simulink model "draft7"  (R2023a)
settings: Solver=VariableStepAuto  StartTime=0.0  StopTime=10  FixedStep=0.0001  MaxStep=0.1  RelTol=1e-3  AbsTol=1e-3  EnableMultiTasking=on
model workspace (MAT data in the model file):
  C_Gimbal = 0.1
  C_IAP = 0.01
  IAP_Pa = 0
  K_Gimbal = 0
  K_IAP = 10
  LeftAbdominalMuscleForce = 0
  LeftBackMuscleForce = 0
  LeftTransverse1MuscleForce = 0
  LeftTransverse2MuscleForce = 0
  Moment_AR = 0
  Moment_FE = 0
  Moment_LB = 0
  RightAbdominalMuscleForce = 0
  RightBackMuscleForce = 0
  RightTransverse1MuscleForce = 0
  RightTransverse2MuscleForce = 0
  a = 1
  b = 1
undefined symbols (not defined in the file): X, Y, Z
libraries: sm_lib x279, nesl_utility x233, simulink_extras x33, checkpacklib x3, simulink x1
(part 5 of 7)

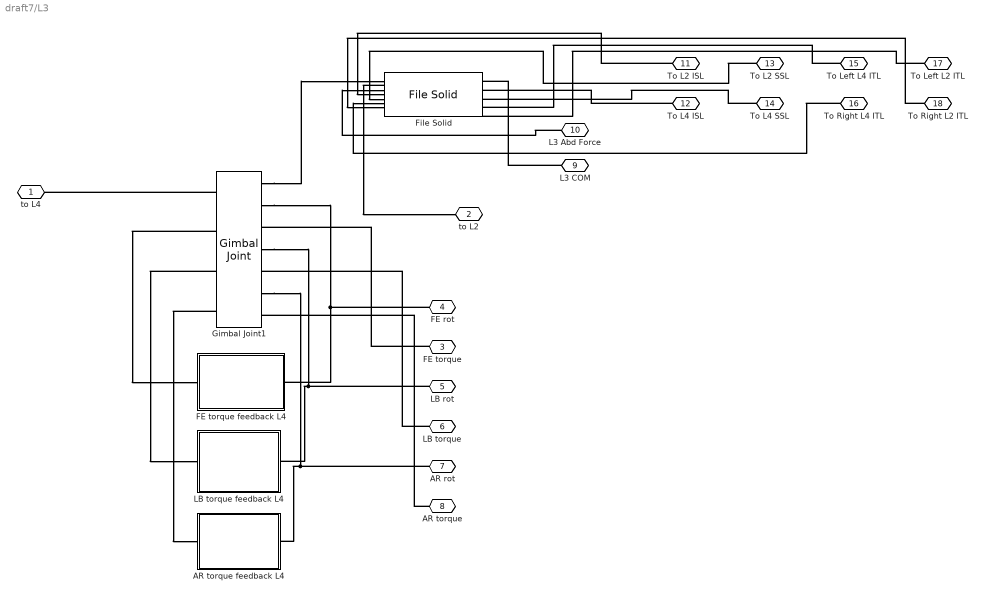
== system draft7/L3 ==
  AR torque feedback L4 : Subsystem
  FE torque feedback L4 : Subsystem
  File Solid : sm_lib/Body Elements/File Solid  ExtGeomFileName=C:\Users\siril\OneDrive\Desktop\TIM-Control\Matlab\Simscape models\CAD - with COM\SymmetricModel\draft7\L3.step  UnitType=FromFile  ExtGeomFileUnits=m  StepReaderType=HEX  ExportConvexHullGeometry=off  InertiaType=CalculateFromGeometry  Mass=1  MassUnits=kg  CenterOfMass=[0 0 0]  CenterOfMassUnits=m  MomentsOfInertia=[1 1 1]  MomentsOfInertiaUnits=kg*m^2  ProductsOfInertia=[0 0 0]  ProductsOfInertiaUnits=kg*m^2  BasedOnType=Density  Density=0.182  DensityUnits=g/cm^3  DoExposeReferenceFrame=on  SerializedFrames=<Frames><Frame><Id>Frame1</Id><Value><Name>To L4</Name><Origin><Source>GeometricFeature</Source><FeatureName>planar surface 3165</FeatureName></Origin><PrimaryAxis><DefinedDirection>+Z</DefinedDirection><Source>GeometricFeature</Source><SourceDirection>+Z</SourceDirection><FeatureName>planar surface 3165</FeatureName></PrimaryAxis><SecondaryAxis><DefinedDirection>+X</DefinedDirection><Source>ReferenceFrame</Source><SourceDirection>+X</SourceDirection><FeatureName></FeatureName></SecondaryAxis></Value></Frame><Frame><Id>Frame2</Id><Value><Name>To L2</Name><Origin><Source>GeometricFeature</Source><FeatureName>planar surface 3181</FeatureName></Origin><PrimaryAxis><DefinedDirection>+Z</DefinedDirection><Source>GeometricFeature</Source><SourceDirection>+Z</SourceDirection><FeatureName>planar surface 3181</FeatureName></PrimaryAxis><SecondaryAxis><DefinedDirection>+X</DefinedDirection><Source>ReferenceFrame</Source><SourceDirection>+X</SourceDirection><FeatureName></FeatureName></SecondaryAxis></Value></Frame><Frame><Id>Frame3</Id><Value><Name>L3 COM</Name><Origin><Source>CenterOfMassFrame</Source><FeatureName></FeatureName></Origin><PrimaryAxis><DefinedDirection>+Z</DefinedDirection><Source>ReferenceFrame</Source><SourceDirection>+Z</SourceDirection><FeatureName></FeatureName></PrimaryAxis><SecondaryAxis><DefinedDirection>+X</DefinedDirection><Source>ReferenceFrame</Source><SourceDirection>+X</SourceDirection><FeatureName></FeatureName></SecondaryAxis></Value></Frame><Frame><Id>Frame4</Id><Value><Name>L3 Abd Force</Name><Origin><Source>GeometricFeature</Source><FeatureName>point 3</FeatureName></Origin><PrimaryAxis><DefinedDirection>+Z</DefinedDirection><Source>GeometricFeature</Source><SourceDirection>+Z</SourceDirection><FeatureName>conical surface 2</FeatureName></PrimaryAxis><SecondaryAxis><DefinedDirection>+X</DefinedDirection><Source>ReferenceFrame</Source><SourceDirection>+X</SourceDirection><FeatureName></FeatureName></SecondaryAxis></Value></Frame><Frame><Id>Frame5</Id><Value><Name>To L4 ISL</Name><Origin><Source>GeometricFeature</Source><FeatureName>point 6019</FeatureName></Origin><PrimaryAxis><DefinedDirection>+Z</DefinedDirection><Source>ReferenceFrame</Source><SourceDirection>+Z</SourceDirection><FeatureName></FeatureName></PrimaryAxis><SecondaryAxis><DefinedDirection>+X</DefinedDirection><Source>ReferenceFrame</Source><SourceDirection>+X</SourceDirection><FeatureName></FeatureName></SecondaryAxis></Value></Frame><Frame><Id>Frame6</Id><Value><Name>To L2 ISL</Name><Origin><Source>GeometricFeature</Source><FeatureName>segment 2486</FeatureName></Origin><PrimaryAxis><DefinedDirection>+Z</DefinedDirection><Source>ReferenceFrame</Source><SourceDirection>+Z</SourceDirection><FeatureName></FeatureName></PrimaryAxis><SecondaryAxis><DefinedDirection>+X</DefinedDirection><Source>ReferenceFrame</Source><SourceDirection>+X</SourceDirection><FeatureName></FeatureName></SecondaryAxis></Value></Frame><Frame><Id>Frame7</Id><Value><Name>To L4 SSL</Name><Origin><Source>GeometricFeature</Source><FeatureName>point 5053</FeatureName></Origin><PrimaryAxis><DefinedDirection>+Z</DefinedDirection><Source>ReferenceFrame</Source><SourceDirection>+Z</SourceDirection><FeatureName></FeatureName></PrimaryAxis><SecondaryAxis><DefinedDirection>+X</DefinedDirection><Source>ReferenceFrame</Source><SourceDirection>+X</SourceDirection><FeatureName></FeatureName></SecondaryAxis></Value></Frame><Frame><Id>Frame8</Id><Value><Name>To L2 SSL</Name><Origin><Source>GeometricFeature</Source><FeatureName>point 5046</FeatureName></Origin><PrimaryAxis><DefinedDirection>+Z</DefinedDirection><Source>ReferenceFrame</Source><SourceDirection>+Z</SourceDirection><FeatureName></FeatureName></PrimaryAxis><SecondaryAxis><DefinedDirection>+X</DefinedDirection><Source>ReferenceFrame</Source><SourceDirection>+X</SourceDirection><FeatureName></FeatureName></SecondaryAxis></Value></Frame><Frame><Id>Frame9</Id><Value><Name>To Left L4 ITL</Name><Origin><Source>GeometricFeature</Source><FeatureName>segment 3930</FeatureName></Origin><PrimaryAxis><DefinedDirection>+Z</DefinedDirection><Source>ReferenceFrame</Source><SourceDirection>+Z</SourceDirection><FeatureName></FeatureName></PrimaryAxis><SecondaryAxis><DefinedDirection>+X</DefinedDirection><Source>ReferenceFrame</Source><SourceDirection>+X</SourceDirection><FeatureName></FeatureName></SecondaryAxis></Value></Frame><Frame><Id>Frame10</Id><Value><Name>To Right L4 ITL</Name><Origin><Source>GeometricFeature</Source><FeatureName>segment 1476</FeatureName></Origin><PrimaryAxis><DefinedDirection>+Z</DefinedDirection><Source>ReferenceFrame</Source><SourceDirection>+Z</SourceDirection><FeatureName></FeatureName></PrimaryAxis><SecondaryAxis><DefinedDirection>+X</DefinedDirection><Source>ReferenceFrame</Source><SourceDirection>+X</SourceDirection><FeatureName></FeatureName></SecondaryAxis></Value></Frame><Frame><Id>Frame11</Id><Value><Name>To Left L2 ITL</Name><Origin><Source>GeometricFeature</Source><FeatureName>point 9469</FeatureName></Origin><PrimaryAxis><DefinedDirection>+Z</DefinedDirection><Source>ReferenceFrame</Source><SourceDirection>+Z</SourceDirection><FeatureName></FeatureName></PrimaryAxis><SecondaryAxis><DefinedDirection>+X</DefinedDirection><Source>ReferenceFrame</Source><SourceDirection>+X</SourceDirection><FeatureName></FeatureName></SecondaryAxis></Value></Frame><Frame><Id>Frame12</Id><Value><Name>To Right L2 ITL</Name><Origin><Source>GeometricFeature</Source><FeatureName>point 3646</FeatureName></Origin><PrimaryAxis><DefinedDirection>+Z</DefinedDirection><Source>ReferenceFrame</Source><SourceDirection>+Z</SourceDirection><FeatureName></FeatureName></PrimaryAxis><SecondaryAxis><DefinedDirection>+X</DefinedDirection><Source>ReferenceFrame</Source><SourceDirection>+X</SourceDirection><FeatureName></FeatureName></SecondaryAxis></Value></Frame></Frames>  GraphicType=FromGeometry  MarkerShape=Sphere  MarkerSize=10  GraphicVisPropType=SimpleVisualProperties  GraphicDiffuseColor=[0.5 0.5 0.5]  GraphicSpecularColor=[0.5 0.5 0.5 1.0]  GraphicAmbientColor=[0.15 0.15 0.15 1.0]  GraphicEmissiveColor=[0.0 0.0 0.0 1.0]  GraphicShininess=75  GraphicOpacity=1.0
  Gimbal Joint1 : sm_lib/Joints/Gimbal Joint  JointMode=Normal  SenseConstraintForce=off  SenseConstraintForceX=off  SenseConstraintForceY=off  SenseConstraintForceZ=off  SenseConstraintTorque=off  SenseConstraintTorqueX=off  SenseConstraintTorqueY=off  SenseConstraintTorqueZ=off  SenseTotalForce=off  SenseTotalForceX=off  SenseTotalForceY=off  SenseTotalForceZ=off  SenseTotalTorque=off  SenseTotalTorqueX=off  SenseTotalTorqueY=off  SenseTotalTorqueZ=off  CompositeWrenchDir=FollowerOnBase  CompositeWrenchFrame=BaseFrame  RxEquilibriumPosition=0  RxEquilibriumPositionUnits=deg  RxSpringStiffness=K_Gimbal  RxSpringStiffnessUnits=N*m/deg  RxDampingCoefficient=C_Gimbal  RxDampingCoefficientUnits=N*m/(deg/s)  RxTorqueActuationMode=InputTorque  RxMotionActuationMode=ComputedMotion  RxSensePosition=on  RxSenseVelocity=off  RxSenseAcceleration=off  RxSenseTorqueForce=on  RxSenseLowerLimitTorqueForce=off  RxSenseUpperLimitTorqueForce=off  RxLowerLimitSpecify=on  RxLowerLimitBound=-30  RxLowerLimitBoundUnits=deg  RxLowerLimitStiffness=10000  RxLowerLimitStiffnessUnits=N*m/deg  RxLowerLimitDamping=100  RxLowerLimitDampingUnits=N*m/(deg/s)  RxLowerLimitTransitionRegionWidth=0.1  RxLowerLimitTransitionRegionWidthUnits=deg  RxUpperLimitSpecify=on  RxUpperLimitBound=30  RxUpperLimitBoundUnits=deg  RxUpperLimitStiffness=10000  RxUpperLimitStiffnessUnits=N*m/deg  RxUpperLimitDamping=100  RxUpperLimitDampingUnits=N*m/(deg/s)  RxUpperLimitTransitionRegionWidth=0.1  RxUpperLimitTransitionRegionWidthUnits=deg  RxPositionTargetSpecify=off  RxPositionTargetPriority=High  RxPositionTargetValue=0  RxPositionTargetValueUnits=deg  RxVelocityTargetSpecify=off  RxVelocityTargetPriority=High  RxVelocityTargetValue=0  RxVelocityTargetValueUnits=deg/s  RyEquilibriumPosition=0  RyEquilibriumPositionUnits=deg  RySpringStiffness=K_Gimbal  RySpringStiffnessUnits=N*m/deg  RyDampingCoefficient=C_Gimbal  RyDampingCoefficientUnits=N*m/(deg/s)  RyTorqueActuationMode=InputTorque  RyMotionActuationMode=ComputedMotion  RySensePosition=on  RySenseVelocity=off  RySenseAcceleration=off  RySenseTorqueForce=on  RySenseLowerLimitTorqueForce=off  RySenseUpperLimitTorqueForce=off  RyLowerLimitSpecify=on  RyLowerLimitBound=-30  RyLowerLimitBoundUnits=deg  RyLowerLimitStiffness=10000  RyLowerLimitStiffnessUnits=N*m/deg  RyLowerLimitDamping=100  RyLowerLimitDampingUnits=N*m/(deg/s)  RyLowerLimitTransitionRegionWidth=0.1  RyLowerLimitTransitionRegionWidthUnits=deg  RyUpperLimitSpecify=on  RyUpperLimitBound=30  RyUpperLimitBoundUnits=deg  RyUpperLimitStiffness=10000  RyUpperLimitStiffnessUnits=N*m/deg  RyUpperLimitDamping=100  RyUpperLimitDampingUnits=N*m/(deg/s)  RyUpperLimitTransitionRegionWidth=0.1  RyUpperLimitTransitionRegionWidthUnits=deg  RyPositionTargetSpecify=off  RyPositionTargetPriority=High  RyPositionTargetValue=0  RyPositionTargetValueUnits=deg  RyVelocityTargetSpecify=off  RyVelocityTargetPriority=High  RyVelocityTargetValue=0  RyVelocityTargetValueUnits=deg/s  RzEquilibriumPosition=0  RzEquilibriumPositionUnits=deg  RzSpringStiffness=K_Gimbal  RzSpringStiffnessUnits=N*m/deg  RzDampingCoefficient=C_Gimbal  RzDampingCoefficientUnits=N*m/(deg/s)  RzTorqueActuationMode=InputTorque  RzMotionActuationMode=ComputedMotion  RzSensePosition=on  RzSenseVelocity=off  RzSenseAcceleration=off  RzSenseTorqueForce=on  RzSenseLowerLimitTorqueForce=off  RzSenseUpperLimitTorqueForce=off  RzLowerLimitSpecify=on  RzLowerLimitBound=-30  RzLowerLimitBoundUnits=deg  RzLowerLimitStiffness=10000  RzLowerLimitStiffnessUnits=N*m/deg  RzLowerLimitDamping=100  RzLowerLimitDampingUnits=N*m/(deg/s)  RzLowerLimitTransitionRegionWidth=0.1  RzLowerLimitTransitionRegionWidthUnits=deg  RzUpperLimitSpecify=on  RzUpperLimitBound=30  RzUpperLimitBoundUnits=deg  RzUpperLimitStiffness=10000  RzUpperLimitStiffnessUnits=N*m/deg  RzUpperLimitDamping=100  RzUpperLimitDampingUnits=N*m/(deg/s)  RzUpperLimitTransitionRegionWidth=0.1  RzUpperLimitTransitionRegionWidthUnits=deg  RzPositionTargetSpecify=off  RzPositionTargetPriority=High  RzPositionTargetValue=0  RzPositionTargetValueUnits=deg  RzVelocityTargetSpecify=off  RzVelocityTargetPriority=High  RzVelocityTargetValue=0  RzVelocityTargetValueUnits=deg/s
  LB torque feedback L4 : Subsystem
  to L4 : PMIOPort  Side=Left
  to L2 : PMIOPort  Port=2  Side=Right
  FE torque : PMIOPort  Port=3  Side=Right
  FE rot : PMIOPort  Port=4  Side=Right
  LB rot : PMIOPort  Port=5  Side=Right
  LB torque : PMIOPort  Port=6  Side=Right
  AR rot : PMIOPort  Port=7  Side=Right
  AR torque : PMIOPort  Port=8  Side=Right
  L3 COM : PMIOPort  Port=9  Side=Right
  L3 Abd Force : PMIOPort  Port=10  Side=Right
  To L2 ISL : PMIOPort  Port=11  Side=Right
  To L4 ISL : PMIOPort  Port=12  Side=Right
  To L2 SSL : PMIOPort  Port=13  Side=Right
  To L4 SSL : PMIOPort  Port=14  Side=Right
  To Left L4 ITL : PMIOPort  Port=15  Side=Right
  To Right L4 ITL : PMIOPort  Port=16  Side=Right
  To Left L2 ITL : PMIOPort  Port=17  Side=Right
  To Right L2 ITL : PMIOPort  Port=18  Side=Right
  connections:
  Gimbal Joint1/LConn1 -- to L4/RConn1
  File Solid/LConn2 -- to L2/RConn1
  Gimbal Joint1/RConn1 -- File Solid/LConn1
  Gimbal Joint1/RConn2 -- FE rot/RConn1 -- FE torque feedback L4/LConn1
  Gimbal Joint1/LConn2 -- FE torque feedback L4/RConn1
  Gimbal Joint1/LConn3 -- LB torque feedback L4/RConn1
  Gimbal Joint1/LConn4 -- AR torque feedback L4/RConn1
  Gimbal Joint1/RConn4 -- LB torque feedback L4/LConn1 -- LB rot/RConn1
  Gimbal Joint1/RConn6 -- AR torque feedback L4/LConn1 -- AR rot/RConn1
  FE torque/RConn1 -- Gimbal Joint1/RConn3
  LB torque/RConn1 -- Gimbal Joint1/RConn5
  AR torque/RConn1 -- Gimbal Joint1/RConn7
  L3 COM/RConn1 -- File Solid/RConn2
  L3 Abd Force/RConn1 -- File Solid/LConn3
  To L4 ISL/RConn1 -- File Solid/RConn3
  To L2 ISL/RConn1 -- File Solid/LConn4
  To L2 SSL/RConn1 -- File Solid/LConn5
  To L4 SSL/RConn1 -- File Solid/RConn4
  To Left L4 ITL/RConn1 -- File Solid/RConn5
  To Right L4 ITL/RConn1 -- File Solid/LConn6
  To Left L2 ITL/RConn1 -- File Solid/RConn6
  To Right L2 ITL/RConn1 -- File Solid/LConn7

== system draft7/L3-L4 AR ==
  Gain3 : Gain  Gain=-1
  Gain8 : Gain
  L3-L4 AR Simscape : Record  FileSettingsInternal="{\"entries\":[{\"content\":{\"excelSettings\":{\"content\":{},\"type\":\"Streamout.ExcelSettings\"}},\"type\":\"Streamout.FileSettingStorage\",\"uuid\":\"23670f92-5bf3-4854-bfd9-fef59633e100\"}],\"packageUris\":[\"http://schema.mathworks.com/mf0/streamout_blocks/R2020a\"],\"version\":\"1.0\"}"  Layout=[1 1]  SignalsInternal="{\"entries\":[{\"content\":{\"signals\":[{\"content\":{\"blockPath\":[\"draft7/L3-L4 AR/L3-L4 AR Simscape\"],\"dimensions\":[1],\"domain\":\"draft7/L3-L4 AR/L3-L4 AR Simscape\",\"lineColor\":\"#edb120\",\"port\":1,\"sid\":[\"\"],\"signalID\":243,\"signalName\":\"L3-L4 AR Simscape Rotation\"},\"type\":\"RecordBlkView.Signal\",\"uuid\":\"bdce66d9-8b2e-421d-9254-30f75ac922b2\"},{\"content\":{\"blockPath\":[\"draft7/L3-L4 AR/L3-L4 AR Simscape\"],\"dimensions\":[1],\"domain\":\"draft7/L3-L4 AR/L3-L4 AR Simscape\",\"lineColor\":\"#7e2f8e\",\"port\":2,\"sid\":[\"\"],\"signalID\":247,\"signalName\":\"L3-L4 AR Simscape Moment\"},\"type\":\"RecordBlkView.Signal\",\"uuid\":\"7bffc420-cc5b-427e-8344-23410ddc9a7b\"}]},\"type\":\"RecordBlkView.InputSignals\",\"uuid\":\"ccd52d68-ef2f-4612-8126-86d92f45f20b\"}],\"packageUris\":[\"http://schema.mathworks.com/mf0/streamout_blocks/R2020a\"],\"version\":\"1.0\"}"  VisualizationBindings="{\"xyplotplugin\":{\"info\":[{\"series\":[],\"subplotID\":1}]}}"  CompatibilityTag=XY
  PS-Simulink Converter : nesl_utility/PS-Simulink Converter  PhysicalDomain=network_engine_domain  SubClassName=ps_output  LeftPortType=input  RightPortType=output  PseudoPeriodic=off  Frequencies=[]  VectorFormat=1-D array  Unit=rad  AffineConversion=off
  PS-Simulink Converter7 : nesl_utility/PS-Simulink Converter  PhysicalDomain=network_engine_domain  SubClassName=ps_output  LeftPortType=input  RightPortType=output  PseudoPeriodic=off  Frequencies=[]  VectorFormat=1-D array  Unit=N*m  AffineConversion=off
  Radians to Degrees : simulink_extras/Transformations/Radians to Degrees
  Scope10 : Scope
  Scope11 : Scope
  Moment : PMIOPort  Side=Left
  Rotation : PMIOPort  Port=2  Side=Left
  wires:
  Radians to Degrees/1 -> Gain3/1
  Gain8/1 -> L3-L4 AR Simscape/2, Scope11/1  "L3-L4 AR Simscape Moment"
  Gain3/1 -> L3-L4 AR Simscape/1, Scope10/1  "L3-L4 AR Simscape Rotation"
  PS-Simulink Converter/1 -> Radians to Degrees/1
  PS-Simulink Converter7/1 -> Gain8/1
  connections:
  Rotation/RConn1 -- PS-Simulink Converter/LConn1
  Moment/RConn1 -- PS-Simulink Converter7/LConn1

== system draft7/L3-L4 FE ==
  Gain3 : Gain  Gain=-1
  Gain8 : Gain
  L3-L4 FE Simscape : Record  FileSettingsInternal="{\"entries\":[{\"content\":{\"excelSettings\":{\"content\":{},\"type\":\"Streamout.ExcelSettings\"}},\"type\":\"Streamout.FileSettingStorage\",\"uuid\":\"aefba751-7f1e-4b9a-a4d5-db69c620bec5\"}],\"packageUris\":[\"http://schema.mathworks.com/mf0/streamout_blocks/R2020a\"],\"version\":\"1.0\"}"  Layout=[1 1]  SignalsInternal="{\"entries\":[{\"content\":{\"signals\":[{\"content\":{\"blockPath\":[\"draft7/L3-L4 FE/L3-L4 FE Simscape\"],\"dimensions\":[1],\"domain\":\"draft7/L3-L4 FE/L3-L4 FE Simscape\",\"lineColor\":\"#77ac30\",\"port\":1,\"sid\":[\"\"],\"signalID\":251,\"signalName\":\"L3-L4 FE Simscape Rotation\"},\"type\":\"RecordBlkView.Signal\",\"uuid\":\"2b32c90d-c1cb-4b03-8021-ce1634e02e03\"},{\"content\":{\"blockPath\":[\"draft7/L3-L4 FE/L3-L4 FE Simscape\"],\"dimensions\":[1],\"domain\":\"draft7/L3-L4 FE/L3-L4 FE Simscape\",\"lineColor\":\"#4dbeee\",\"port\":2,\"sid\":[\"\"],\"signalID\":255,\"signalName\":\"L3-L4 FE Simscape Moment\"},\"type\":\"RecordBlkView.Signal\",\"uuid\":\"7fa56d1d-9083-47ad-a9f3-aca98951c653\"}]},\"type\":\"RecordBlkView.InputSignals\",\"uuid\":\"07111957-07c9-4499-bcc7-35cf704713cb\"}],\"packageUris\":[\"http://schema.mathworks.com/mf0/streamout_blocks/R2020a\"],\"version\":\"1.0\"}"  VisualizationBindings="{\"xyplotplugin\":{\"info\":[{\"series\":[],\"subplotID\":1}]}}"  CompatibilityTag=XY
  PS-Simulink Converter : nesl_utility/PS-Simulink Converter  PhysicalDomain=network_engine_domain  SubClassName=ps_output  LeftPortType=input  RightPortType=output  PseudoPeriodic=off  Frequencies=[]  VectorFormat=1-D array  Unit=rad  AffineConversion=off
  PS-Simulink Converter7 : nesl_utility/PS-Simulink Converter  PhysicalDomain=network_engine_domain  SubClassName=ps_output  LeftPortType=input  RightPortType=output  PseudoPeriodic=off  Frequencies=[]  VectorFormat=1-D array  Unit=N*m  AffineConversion=off
  Radians to Degrees : simulink_extras/Transformations/Radians to Degrees
  Scope10 : Scope
  Scope11 : Scope
  Moment : PMIOPort  Side=Left
  Rotation : PMIOPort  Port=2  Side=Left
  wires:
  Radians to Degrees/1 -> Gain3/1
  Gain8/1 -> L3-L4 FE Simscape/2, Scope11/1  "L3-L4 FE Simscape Moment"
  Gain3/1 -> L3-L4 FE Simscape/1, Scope10/1  "L3-L4 FE Simscape Rotation"
  PS-Simulink Converter/1 -> Radians to Degrees/1
  PS-Simulink Converter7/1 -> Gain8/1
  connections:
  Rotation/RConn1 -- PS-Simulink Converter/LConn1
  Moment/RConn1 -- PS-Simulink Converter7/LConn1

== system draft7/L3-L4 LB ==
  Gain3 : Gain
  Gain8 : Gain  Gain=-1
  L3-L4 LB Simscape : Record  FileSettingsInternal="{\"entries\":[{\"content\":{\"excelSettings\":{\"content\":{},\"type\":\"Streamout.ExcelSettings\"}},\"type\":\"Streamout.FileSettingStorage\",\"uuid\":\"1b8c23e1-381b-441a-8fd2-30b648a111b9\"}],\"packageUris\":[\"http://schema.mathworks.com/mf0/streamout_blocks/R2020a\"],\"version\":\"1.0\"}"  Layout=[1 1]  SignalsInternal="{\"entries\":[{\"content\":{\"signals\":[{\"content\":{\"blockPath\":[\"draft7/L3-L4 LB/L3-L4 LB Simscape\"],\"dimensions\":[1],\"domain\":\"draft7/L3-L4 LB/L3-L4 LB Simscape\",\"lineColor\":\"#a2142f\",\"port\":1,\"sid\":[\"\"],\"signalID\":259,\"signalName\":\"L3-L4 LB Simscape Rotation\"},\"type\":\"RecordBlkView.Signal\",\"uuid\":\"1b9f3bf6-4b2a-4b6d-8cc4-964c709bb45b\"},{\"content\":{\"blockPath\":[\"draft7/L3-L4 LB/L3-L4 LB Simscape\"],\"dimensions\":[1],\"domain\":\"draft7/L3-L4 LB/L3-L4 LB Simscape\",\"lineColor\":\"#139fff\",\"port\":2,\"sid\":[\"\"],\"signalID\":263,\"signalName\":\"L3-L4 LB Simscape Moment\"},\"type\":\"RecordBlkView.Signal\",\"uuid\":\"4da0e45f-f007-4264-93d6-83f55e9e681e\"}]},\"type\":\"RecordBlkView.InputSignals\",\"uuid\":\"90bf3f15-ea2c-4759-89a9-3907d0708b4c\"}],\"packageUris\":[\"http://schema.mathworks.com/mf0/streamout_blocks/R2020a\"],\"version\":\"1.0\"}"  VisualizationBindings="{\"xyplotplugin\":{\"info\":[{\"series\":[],\"subplotID\":1}]}}"  CompatibilityTag=XY
  PS-Simulink Converter : nesl_utility/PS-Simulink Converter  PhysicalDomain=network_engine_domain  SubClassName=ps_output  LeftPortType=input  RightPortType=output  PseudoPeriodic=off  Frequencies=[]  VectorFormat=1-D array  Unit=rad  AffineConversion=off
  PS-Simulink Converter7 : nesl_utility/PS-Simulink Converter  PhysicalDomain=network_engine_domain  SubClassName=ps_output  LeftPortType=input  RightPortType=output  PseudoPeriodic=off  Frequencies=[]  VectorFormat=1-D array  Unit=N*m  AffineConversion=off
  Radians to Degrees : simulink_extras/Transformations/Radians to Degrees
  Scope10 : Scope
  Scope11 : Scope
  Moment : PMIOPort  Side=Left
  Rotation : PMIOPort  Port=2  Side=Left
  wires:
  Radians to Degrees/1 -> Gain3/1
  Gain8/1 -> L3-L4 LB Simscape/2, Scope11/1  "L3-L4 LB Simscape Moment"
  Gain3/1 -> L3-L4 LB Simscape/1, Scope10/1  "L3-L4 LB Simscape Rotation"
  PS-Simulink Converter/1 -> Radians to Degrees/1
  PS-Simulink Converter7/1 -> Gain8/1
  connections:
  Rotation/RConn1 -- PS-Simulink Converter/LConn1
  Moment/RConn1 -- PS-Simulink Converter7/LConn1

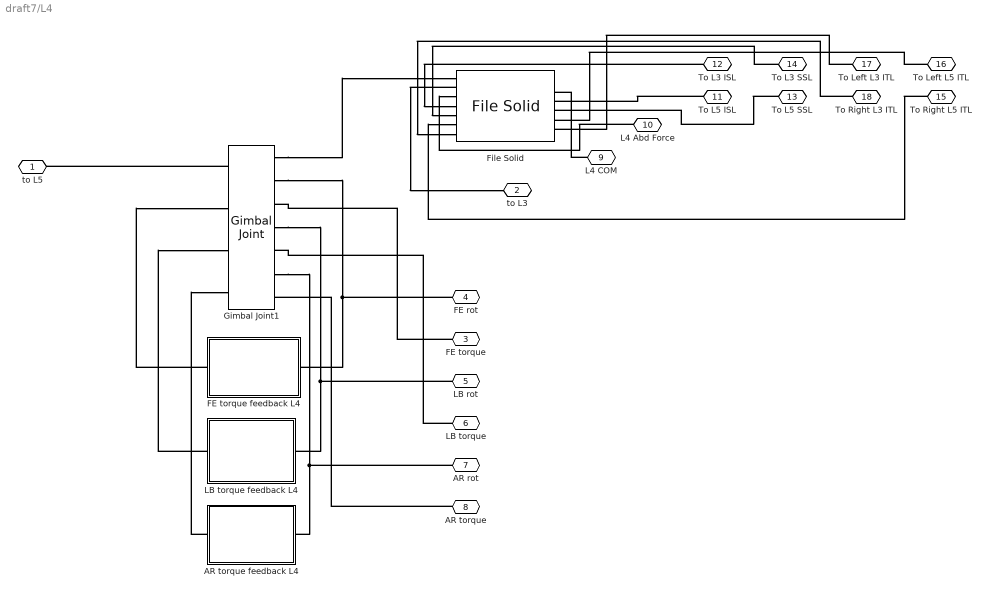
== system draft7/L4 ==
  AR torque feedback L4 : Subsystem
  FE torque feedback L4 : Subsystem
  File Solid : sm_lib/Body Elements/File Solid  ExtGeomFileName=C:\Users\siril\OneDrive\Desktop\TIM-Control\Matlab\Simscape models\CAD - with COM\SymmetricModel\draft7\L4.step  UnitType=FromFile  ExtGeomFileUnits=m  StepReaderType=HEX  ExportConvexHullGeometry=off  InertiaType=CalculateFromGeometry  Mass=1  MassUnits=kg  CenterOfMass=[0 0 0]  CenterOfMassUnits=m  MomentsOfInertia=[1 1 1]  MomentsOfInertiaUnits=kg*m^2  ProductsOfInertia=[0 0 0]  ProductsOfInertiaUnits=kg*m^2  BasedOnType=Density  Density=0.182  DensityUnits=g/cm^3  DoExposeReferenceFrame=on  SerializedFrames=<Frames><Frame><Id>Frame1</Id><Value><Name>To L5</Name><Origin><Source>GeometricFeature</Source><FeatureName>planar surface 3686</FeatureName></Origin><PrimaryAxis><DefinedDirection>+Z</DefinedDirection><Source>GeometricFeature</Source><SourceDirection>+Z</SourceDirection><FeatureName>planar surface 3686</FeatureName></PrimaryAxis><SecondaryAxis><DefinedDirection>+X</DefinedDirection><Source>ReferenceFrame</Source><SourceDirection>+X</SourceDirection><FeatureName></FeatureName></SecondaryAxis></Value></Frame><Frame><Id>Frame2</Id><Value><Name>To L3</Name><Origin><Source>GeometricFeature</Source><FeatureName>planar surface 3752</FeatureName></Origin><PrimaryAxis><DefinedDirection>+Z</DefinedDirection><Source>GeometricFeature</Source><SourceDirection>+Z</SourceDirection><FeatureName>planar surface 3752</FeatureName></PrimaryAxis><SecondaryAxis><DefinedDirection>+X</DefinedDirection><Source>ReferenceFrame</Source><SourceDirection>+X</SourceDirection><FeatureName></FeatureName></SecondaryAxis></Value></Frame><Frame><Id>Frame3</Id><Value><Name>L4 COM</Name><Origin><Source>CenterOfMassFrame</Source><FeatureName></FeatureName></Origin><PrimaryAxis><DefinedDirection>+Z</DefinedDirection><Source>ReferenceFrame</Source><SourceDirection>+Z</SourceDirection><FeatureName></FeatureName></PrimaryAxis><SecondaryAxis><DefinedDirection>+X</DefinedDirection><Source>ReferenceFrame</Source><SourceDirection>+X</SourceDirection><FeatureName></FeatureName></SecondaryAxis></Value></Frame><Frame><Id>Frame4</Id><Value><Name>L4 Abd Force</Name><Origin><Source>GeometricFeature</Source><FeatureName>point 3</FeatureName></Origin><PrimaryAxis><DefinedDirection>+Z</DefinedDirection><Source>GeometricFeature</Source><SourceDirection>+Z</SourceDirection><FeatureName>conical surface 2</FeatureName></PrimaryAxis><SecondaryAxis><DefinedDirection>+X</DefinedDirection><Source>ReferenceFrame</Source><SourceDirection>+X</SourceDirection><FeatureName></FeatureName></SecondaryAxis></Value></Frame><Frame><Id>Frame5</Id><Value><Name>To L5 ISL</Name><Origin><Source>GeometricFeature</Source><FeatureName>point 5953</FeatureName></Origin><PrimaryAxis><DefinedDirection>+Z</DefinedDirection><Source>ReferenceFrame</Source><SourceDirection>+Z</SourceDirection><FeatureName></FeatureName></PrimaryAxis><SecondaryAxis><DefinedDirection>+X</DefinedDirection><Source>ReferenceFrame</Source><SourceDirection>+X</SourceDirection><FeatureName></FeatureName></SecondaryAxis></Value></Frame><Frame><Id>Frame6</Id><Value><Name>To L3 ISL</Name><Origin><Source>GeometricFeature</Source><FeatureName>point 5708</FeatureName></Origin><PrimaryAxis><DefinedDirection>+Z</DefinedDirection><Source>ReferenceFrame</Source><SourceDirection>+Z</SourceDirection><FeatureName></FeatureName></PrimaryAxis><SecondaryAxis><DefinedDirection>+X</DefinedDirection><Source>ReferenceFrame</Source><SourceDirection>+X</SourceDirection><FeatureName></FeatureName></SecondaryAxis></Value></Frame><Frame><Id>Frame7</Id><Value><Name>To L5 SSL</Name><Origin><Source>GeometricFeature</Source><FeatureName>segment 1184</FeatureName></Origin><PrimaryAxis><DefinedDirection>+Z</DefinedDirection><Source>ReferenceFrame</Source><SourceDirection>+Z</SourceDirection><FeatureName></FeatureName></PrimaryAxis><SecondaryAxis><DefinedDirection>+X</DefinedDirection><Source>ReferenceFrame</Source><SourceDirection>+X</SourceDirection><FeatureName></FeatureName></SecondaryAxis></Value></Frame><Frame><Id>Frame8</Id><Value><Name>To L3 SSL</Name><Origin><Source>GeometricFeature</Source><FeatureName>segment 1187</FeatureName></Origin><PrimaryAxis><DefinedDirection>+Z</DefinedDirection><Source>ReferenceFrame</Source><SourceDirection>+Z</SourceDirection><FeatureName></FeatureName></PrimaryAxis><SecondaryAxis><DefinedDirection>+X</DefinedDirection><Source>ReferenceFrame</Source><SourceDirection>+X</SourceDirection><FeatureName></FeatureName></SecondaryAxis></Value></Frame><Frame><Id>Frame9</Id><Value><Name>To Left L5 ITL</Name><Origin><Source>GeometricFeature</Source><FeatureName>segment 5066</FeatureName></Origin><PrimaryAxis><DefinedDirection>+Z</DefinedDirection><Source>ReferenceFrame</Source><SourceDirection>+Z</SourceDirection><FeatureName></FeatureName></PrimaryAxis><SecondaryAxis><DefinedDirection>+X</DefinedDirection><Source>ReferenceFrame</Source><SourceDirection>+X</SourceDirection><FeatureName></FeatureName></SecondaryAxis></Value></Frame><Frame><Id>Frame10</Id><Value><Name>To Right L5 ITL</Name><Origin><Source>GeometricFeature</Source><FeatureName>segment 2206</FeatureName></Origin><PrimaryAxis><DefinedDirection>+Z</DefinedDirection><Source>ReferenceFrame</Source><SourceDirection>+Z</SourceDirection><FeatureName></FeatureName></PrimaryAxis><SecondaryAxis><DefinedDirection>+X</DefinedDirection><Source>ReferenceFrame</Source><SourceDirection>+X</SourceDirection><FeatureName></FeatureName></SecondaryAxis></Value></Frame><Frame><Id>Frame11</Id><Value><Name>To Left L3 ITL</Name><Origin><Source>GeometricFeature</Source><FeatureName>point 10404</FeatureName></Origin><PrimaryAxis><DefinedDirection>+Z</DefinedDirection><Source>ReferenceFrame</Source><SourceDirection>+Z</SourceDirection><FeatureName></FeatureName></PrimaryAxis><SecondaryAxis><DefinedDirection>+X</DefinedDirection><Source>ReferenceFrame</Source><SourceDirection>+X</SourceDirection><FeatureName></FeatureName></SecondaryAxis></Value></Frame><Frame><Id>Frame12</Id><Value><Name>To Right L3 ITL</Name><Origin><Source>GeometricFeature</Source><FeatureName>point 4693</FeatureName></Origin><PrimaryAxis><DefinedDirection>+Z</DefinedDirection><Source>ReferenceFrame</Source><SourceDirection>+Z</SourceDirection><FeatureName></FeatureName></PrimaryAxis><SecondaryAxis><DefinedDirection>+X</DefinedDirection><Source>ReferenceFrame</Source><SourceDirection>+X</SourceDirection><FeatureName></FeatureName></SecondaryAxis></Value></Frame></Frames>  GraphicType=FromGeometry  MarkerShape=Sphere  MarkerSize=10  GraphicVisPropType=SimpleVisualProperties  GraphicDiffuseColor=[0.5 0.5 0.5]  GraphicSpecularColor=[0.5 0.5 0.5 1.0]  GraphicAmbientColor=[0.15 0.15 0.15 1.0]  GraphicEmissiveColor=[0.0 0.0 0.0 1.0]  GraphicShininess=75  GraphicOpacity=1.0
  Gimbal Joint1 : sm_lib/Joints/Gimbal Joint  JointMode=Normal  SenseConstraintForce=off  SenseConstraintForceX=off  SenseConstraintForceY=off  SenseConstraintForceZ=off  SenseConstraintTorque=off  SenseConstraintTorqueX=off  SenseConstraintTorqueY=off  SenseConstraintTorqueZ=off  SenseTotalForce=off  SenseTotalForceX=off  SenseTotalForceY=off  SenseTotalForceZ=off  SenseTotalTorque=off  SenseTotalTorqueX=off  SenseTotalTorqueY=off  SenseTotalTorqueZ=off  CompositeWrenchDir=FollowerOnBase  CompositeWrenchFrame=BaseFrame  RxEquilibriumPosition=0  RxEquilibriumPositionUnits=deg  RxSpringStiffness=K_Gimbal  RxSpringStiffnessUnits=N*m/deg  RxDampingCoefficient=C_Gimbal  RxDampingCoefficientUnits=N*m/(deg/s)  RxTorqueActuationMode=InputTorque  RxMotionActuationMode=ComputedMotion  RxSensePosition=on  RxSenseVelocity=off  RxSenseAcceleration=off  RxSenseTorqueForce=on  RxSenseLowerLimitTorqueForce=off  RxSenseUpperLimitTorqueForce=off  RxLowerLimitSpecify=on  RxLowerLimitBound=-30  RxLowerLimitBoundUnits=deg  RxLowerLimitStiffness=10000  RxLowerLimitStiffnessUnits=N*m/deg  RxLowerLimitDamping=100  RxLowerLimitDampingUnits=N*m/(deg/s)  RxLowerLimitTransitionRegionWidth=0.1  RxLowerLimitTransitionRegionWidthUnits=deg  RxUpperLimitSpecify=on  RxUpperLimitBound=30  RxUpperLimitBoundUnits=deg  RxUpperLimitStiffness=10000  RxUpperLimitStiffnessUnits=N*m/deg  RxUpperLimitDamping=100  RxUpperLimitDampingUnits=N*m/(deg/s)  RxUpperLimitTransitionRegionWidth=0.1  RxUpperLimitTransitionRegionWidthUnits=deg  RxPositionTargetSpecify=off  RxPositionTargetPriority=High  RxPositionTargetValue=0  RxPositionTargetValueUnits=deg  RxVelocityTargetSpecify=off  RxVelocityTargetPriority=High  RxVelocityTargetValue=0  RxVelocityTargetValueUnits=deg/s  RyEquilibriumPosition=0  RyEquilibriumPositionUnits=deg  RySpringStiffness=K_Gimbal  RySpringStiffnessUnits=N*m/deg  RyDampingCoefficient=C_Gimbal  RyDampingCoefficientUnits=N*m/(deg/s)  RyTorqueActuationMode=InputTorque  RyMotionActuationMode=ComputedMotion  RySensePosition=on  RySenseVelocity=off  RySenseAcceleration=off  RySenseTorqueForce=on  RySenseLowerLimitTorqueForce=off  RySenseUpperLimitTorqueForce=off  RyLowerLimitSpecify=on  RyLowerLimitBound=-30  RyLowerLimitBoundUnits=deg  RyLowerLimitStiffness=10000  RyLowerLimitStiffnessUnits=N*m/deg  RyLowerLimitDamping=100  RyLowerLimitDampingUnits=N*m/(deg/s)  RyLowerLimitTransitionRegionWidth=0.1  RyLowerLimitTransitionRegionWidthUnits=deg  RyUpperLimitSpecify=on  RyUpperLimitBound=30  RyUpperLimitBoundUnits=deg  RyUpperLimitStiffness=10000  RyUpperLimitStiffnessUnits=N*m/deg  RyUpperLimitDamping=100  RyUpperLimitDampingUnits=N*m/(deg/s)  RyUpperLimitTransitionRegionWidth=0.1  RyUpperLimitTransitionRegionWidthUnits=deg  RyPositionTargetSpecify=off  RyPositionTargetPriority=High  RyPositionTargetValue=0  RyPositionTargetValueUnits=deg  RyVelocityTargetSpecify=off  RyVelocityTargetPriority=High  RyVelocityTargetValue=0  RyVelocityTargetValueUnits=deg/s  RzEquilibriumPosition=0  RzEquilibriumPositionUnits=deg  RzSpringStiffness=K_Gimbal  RzSpringStiffnessUnits=N*m/deg  RzDampingCoefficient=C_Gimbal  RzDampingCoefficientUnits=N*m/(deg/s)  RzTorqueActuationMode=InputTorque  RzMotionActuationMode=ComputedMotion  RzSensePosition=on  RzSenseVelocity=off  RzSenseAcceleration=off  RzSenseTorqueForce=on  RzSenseLowerLimitTorqueForce=off  RzSenseUpperLimitTorqueForce=off  RzLowerLimitSpecify=on  RzLowerLimitBound=-30  RzLowerLimitBoundUnits=deg  RzLowerLimitStiffness=10000  RzLowerLimitStiffnessUnits=N*m/deg  RzLowerLimitDamping=100  RzLowerLimitDampingUnits=N*m/(deg/s)  RzLowerLimitTransitionRegionWidth=0.1  RzLowerLimitTransitionRegionWidthUnits=deg  RzUpperLimitSpecify=on  RzUpperLimitBound=30  RzUpperLimitBoundUnits=deg  RzUpperLimitStiffness=10000  RzUpperLimitStiffnessUnits=N*m/deg  RzUpperLimitDamping=100  RzUpperLimitDampingUnits=N*m/(deg/s)  RzUpperLimitTransitionRegionWidth=0.1  RzUpperLimitTransitionRegionWidthUnits=deg  RzPositionTargetSpecify=off  RzPositionTargetPriority=High  RzPositionTargetValue=0  RzPositionTargetValueUnits=deg  RzVelocityTargetSpecify=off  RzVelocityTargetPriority=High  RzVelocityTargetValue=0  RzVelocityTargetValueUnits=deg/s
  LB torque feedback L4 : Subsystem
  to L5 : PMIOPort  Side=Left
  to L3 : PMIOPort  Port=2  Side=Right
  FE torque : PMIOPort  Port=3  Side=Right
  FE rot : PMIOPort  Port=4  Side=Right
  LB rot : PMIOPort  Port=5  Side=Right
  LB torque : PMIOPort  Port=6  Side=Right
  AR rot : PMIOPort  Port=7  Side=Right
  AR torque : PMIOPort  Port=8  Side=Right
  L4 COM : PMIOPort  Port=9  Side=Right
  L4 Abd Force : PMIOPort  Port=10  Side=Right
  To L5 ISL : PMIOPort  Port=11  Side=Right
  To L3 ISL : PMIOPort  Port=12  Side=Right
  To L5 SSL : PMIOPort  Port=13  Side=Right
  To L3 SSL : PMIOPort  Port=14  Side=Right
  To Right L5 ITL : PMIOPort  Port=15  Side=Right
  To Left L5 ITL : PMIOPort  Port=16  Side=Right
  To Left L3 ITL : PMIOPort  Port=17  Side=Right
  To Right L3 ITL : PMIOPort  Port=18  Side=Right
  connections:
  Gimbal Joint1/LConn1 -- to L5/RConn1
  File Solid/LConn2 -- to L3/RConn1
  Gimbal Joint1/RConn1 -- File Solid/LConn1
  Gimbal Joint1/RConn2 -- FE rot/RConn1 -- FE torque feedback L4/LConn1
  AR torque feedback L4/RConn1 -- Gimbal Joint1/LConn4
  LB torque feedback L4/RConn1 -- Gimbal Joint1/LConn3
  FE torque feedback L4/RConn1 -- Gimbal Joint1/LConn2
  Gimbal Joint1/RConn4 -- LB rot/RConn1 -- LB torque feedback L4/LConn1
  Gimbal Joint1/RConn6 -- AR rot/RConn1 -- AR torque feedback L4/LConn1
  FE torque/RConn1 -- Gimbal Joint1/RConn3
  LB torque/RConn1 -- Gimbal Joint1/RConn5
  AR torque/RConn1 -- Gimbal Joint1/RConn7
  L4 COM/RConn1 -- File Solid/RConn2
  L4 Abd Force/RConn1 -- File Solid/LConn3
  To L5 ISL/RConn1 -- File Solid/RConn3
  To L3 ISL/RConn1 -- File Solid/LConn4
  To L5 SSL/RConn1 -- File Solid/RConn4
  To L3 SSL/RConn1 -- File Solid/LConn5
  To Left L3 ITL/RConn1 -- File Solid/RConn6
  To Left L5 ITL/RConn1 -- File Solid/RConn5
  To Right L3 ITL/RConn1 -- File Solid/LConn7
  To Right L5 ITL/RConn1 -- File Solid/LConn6

== system draft7/L4-L5  AR ==
  Gain3 : Gain  Gain=-1
  Gain8 : Gain
  L4-L5 AR Simscape : Record  FileSettingsInternal="{\"entries\":[{\"content\":{\"excelSettings\":{\"content\":{},\"type\":\"Streamout.ExcelSettings\"}},\"type\":\"Streamout.FileSettingStorage\",\"uuid\":\"8bbbd22b-107f-4fdb-8523-2e709e31aafd\"}],\"packageUris\":[\"http://schema.mathworks.com/mf0/streamout_blocks/R2020a\"],\"version\":\"1.0\"}"  Layout=[1 1]  SignalsInternal="{\"entries\":[{\"content\":{\"signals\":[{\"content\":{\"blockPath\":[\"draft7/L4-L5  AR/L4-L5 AR Simscape\"],\"dimensions\":[1],\"domain\":\"draft7/L4-L5  AR/L4-L5 AR Simscape\",\"lineColor\":\"#ff6929\",\"port\":1,\"sid\":[\"\"],\"signalID\":267,\"signalName\":\"L4-L5 AR Simscape Rotation\"},\"type\":\"RecordBlkView.Signal\",\"uuid\":\"43c49ab6-926d-450d-9865-27fc7350793f\"},{\"content\":{\"blockPath\":[\"draft7/L4-L5  AR/L4-L5 AR Simscape\"],\"dimensions\":[1],\"domain\":\"draft7/L4-L5  AR/L4-L5 AR Simscape\",\"lineColor\":\"#b746ff\",\"port\":2,\"sid\":[\"\"],\"signalID\":271,\"signalName\":\"L4-L5 AR Simscape Moment\"},\"type\":\"RecordBlkView.Signal\",\"uuid\":\"148edb12-5ddf-4fc6-9b32-e195f22cf50b\"}]},\"type\":\"RecordBlkView.InputSignals\",\"uuid\":\"b60c2a5d-f707-4901-95c8-171bd48b2b76\"}],\"packageUris\":[\"http://schema.mathworks.com/mf0/streamout_blocks/R2020a\"],\"version\":\"1.0\"}"  VisualizationBindings="{\"xyplotplugin\":{\"info\":[{\"series\":[],\"subplotID\":1}]}}"  CompatibilityTag=XY
  PS-Simulink Converter : nesl_utility/PS-Simulink Converter  PhysicalDomain=network_engine_domain  SubClassName=ps_output  LeftPortType=input  RightPortType=output  PseudoPeriodic=off  Frequencies=[]  VectorFormat=1-D array  Unit=rad  AffineConversion=off
  PS-Simulink Converter7 : nesl_utility/PS-Simulink Converter  PhysicalDomain=network_engine_domain  SubClassName=ps_output  LeftPortType=input  RightPortType=output  PseudoPeriodic=off  Frequencies=[]  VectorFormat=1-D array  Unit=N*m  AffineConversion=off
  Radians to Degrees : simulink_extras/Transformations/Radians to Degrees
  Scope10 : Scope
  Scope11 : Scope
  Moment : PMIOPort  Side=Left
  Rotation : PMIOPort  Port=2  Side=Left
  wires:
  Radians to Degrees/1 -> Gain3/1
  Gain8/1 -> L4-L5 AR Simscape/2, Scope11/1  "L4-L5 AR Simscape Moment"
  Gain3/1 -> L4-L5 AR Simscape/1, Scope10/1  "L4-L5 AR Simscape Rotation"
  PS-Simulink Converter/1 -> Radians to Degrees/1
  PS-Simulink Converter7/1 -> Gain8/1
  connections:
  Rotation/RConn1 -- PS-Simulink Converter/LConn1
  Moment/RConn1 -- PS-Simulink Converter7/LConn1

== system draft7/L4-L5  FE ==
  Gain3 : Gain  Gain=-1
  Gain8 : Gain
  L4-L5 FE Simscape : Record  FileSettingsInternal="{\"entries\":[{\"content\":{\"excelSettings\":{\"content\":{},\"type\":\"Streamout.ExcelSettings\"}},\"type\":\"Streamout.FileSettingStorage\",\"uuid\":\"cf3bae49-f78f-4d86-ac5e-3c046f9051ff\"}],\"packageUris\":[\"http://schema.mathworks.com/mf0/streamout_blocks/R2020a\"],\"version\":\"1.0\"}"  Layout=[1 1]  SignalsInternal="{\"entries\":[{\"content\":{\"signals\":[{\"content\":{\"blockPath\":[\"draft7/L4-L5  FE/L4-L5 FE Simscape\"],\"dimensions\":[1],\"domain\":\"draft7/L4-L5  FE/L4-L5 FE Simscape\",\"lineColor\":\"#64d413\",\"port\":1,\"sid\":[\"\"],\"signalID\":275,\"signalName\":\"L4-L5 FE Simscape Rotation\"},\"type\":\"RecordBlkView.Signal\",\"uuid\":\"a1eaf24c-21b6-4e92-aa71-fcfe9f21c4e6\"},{\"content\":{\"blockPath\":[\"draft7/L4-L5  FE/L4-L5 FE Simscape\"],\"dimensions\":[1],\"domain\":\"draft7/L4-L5  FE/L4-L5 FE Simscape\",\"lineColor\":\"#ff13a6\",\"port\":2,\"sid\":[\"\"],\"signalID\":279,\"signalName\":\"L4-L5 FE Simscape Moment\"},\"type\":\"RecordBlkView.Signal\",\"uuid\":\"e6f15731-cd27-4cb6-9084-093c3ee28111\"}]},\"type\":\"RecordBlkView.InputSignals\",\"uuid\":\"8ab26356-5ff2-4ca0-a1a7-af66fb5d6252\"}],\"packageUris\":[\"http://schema.mathworks.com/mf0/streamout_blocks/R2020a\"],\"version\":\"1.0\"}"  VisualizationBindings="{\"xyplotplugin\":{\"info\":[{\"series\":[],\"subplotID\":1}]}}"  CompatibilityTag=XY
  PS-Simulink Converter : nesl_utility/PS-Simulink Converter  PhysicalDomain=network_engine_domain  SubClassName=ps_output  LeftPortType=input  RightPortType=output  PseudoPeriodic=off  Frequencies=[]  VectorFormat=1-D array  Unit=rad  AffineConversion=off
  PS-Simulink Converter7 : nesl_utility/PS-Simulink Converter  PhysicalDomain=network_engine_domain  SubClassName=ps_output  LeftPortType=input  RightPortType=output  PseudoPeriodic=off  Frequencies=[]  VectorFormat=1-D array  Unit=N*m  AffineConversion=off
  Radians to Degrees : simulink_extras/Transformations/Radians to Degrees
  Scope10 : Scope
  Scope11 : Scope
  Moment : PMIOPort  Side=Left
  Rotation : PMIOPort  Port=2  Side=Left
  wires:
  Radians to Degrees/1 -> Gain3/1
  Gain8/1 -> L4-L5 FE Simscape/2, Scope11/1  "L4-L5 FE Simscape Moment"
  Gain3/1 -> L4-L5 FE Simscape/1, Scope10/1  "L4-L5 FE Simscape Rotation"
  PS-Simulink Converter/1 -> Radians to Degrees/1
  PS-Simulink Converter7/1 -> Gain8/1
  connections:
  Rotation/RConn1 -- PS-Simulink Converter/LConn1
  Moment/RConn1 -- PS-Simulink Converter7/LConn1

== system draft7/L4-L5  LB ==
  Gain3 : Gain
  Gain8 : Gain  Gain=-1
  L4-L5 LB Simscape : Record  FileSettingsInternal="{\"entries\":[{\"content\":{\"excelSettings\":{\"content\":{},\"type\":\"Streamout.ExcelSettings\"}},\"type\":\"Streamout.FileSettingStorage\",\"uuid\":\"50bf8c5e-2651-45d7-8a3c-ee0dd698c777\"}],\"packageUris\":[\"http://schema.mathworks.com/mf0/streamout_blocks/R2020a\"],\"version\":\"1.0\"}"  Layout=[1 1]  SignalsInternal="{\"entries\":[{\"content\":{\"signals\":[{\"content\":{\"blockPath\":[\"draft7/L4-L5  LB/L4-L5 LB Simscape\"],\"dimensions\":[1],\"domain\":\"draft7/L4-L5  LB/L4-L5 LB Simscape\",\"lineColor\":\"#fe330a\",\"port\":1,\"sid\":[\"\"],\"signalID\":283,\"signalName\":\"L4-L5 LB Simscape Rotation\"},\"type\":\"RecordBlkView.Signal\",\"uuid\":\"9a47e534-4785-45c9-a01c-416127989aef\"},{\"content\":{\"blockPath\":[\"draft7/L4-L5  LB/L4-L5 LB Simscape\"],\"dimensions\":[1],\"domain\":\"draft7/L4-L5  LB/L4-L5 LB Simscape\",\"lineColor\":\"#22b573\",\"port\":2,\"sid\":[\"\"],\"signalID\":287,\"signalName\":\"L4-L5 LB Simscape Moment\"},\"type\":\"RecordBlkView.Signal\",\"uuid\":\"5e1e194d-d45e-4890-9d68-c2c2ae2c91f1\"}]},\"type\":\"RecordBlkView.InputSignals\",\"uuid\":\"53d82c13-78b0-4212-adb8-598b381078ac\"}],\"packageUris\":[\"http://schema.mathworks.com/mf0/streamout_blocks/R2020a\"],\"version\":\"1.0\"}"  VisualizationBindings="{\"xyplotplugin\":{\"info\":[{\"series\":[],\"subplotID\":1}]}}"  CompatibilityTag=XY
  PS-Simulink Converter : nesl_utility/PS-Simulink Converter  PhysicalDomain=network_engine_domain  SubClassName=ps_output  LeftPortType=input  RightPortType=output  PseudoPeriodic=off  Frequencies=[]  VectorFormat=1-D array  Unit=rad  AffineConversion=off
  PS-Simulink Converter7 : nesl_utility/PS-Simulink Converter  PhysicalDomain=network_engine_domain  SubClassName=ps_output  LeftPortType=input  RightPortType=output  PseudoPeriodic=off  Frequencies=[]  VectorFormat=1-D array  Unit=N*m  AffineConversion=off
  Radians to Degrees : simulink_extras/Transformations/Radians to Degrees
  Scope10 : Scope
  Scope11 : Scope
  Moment : PMIOPort  Side=Left
  Rotation : PMIOPort  Port=2  Side=Left
  wires:
  Radians to Degrees/1 -> Gain3/1
  Gain8/1 -> L4-L5 LB Simscape/2, Scope11/1  "L4-L5 LB Simscape Moment"
  Gain3/1 -> L4-L5 LB Simscape/1, Scope10/1  "L4-L5 LB Simscape Rotation"
  PS-Simulink Converter/1 -> Radians to Degrees/1
  PS-Simulink Converter7/1 -> Gain8/1
  connections:
  Rotation/RConn1 -- PS-Simulink Converter/LConn1
  Moment/RConn1 -- PS-Simulink Converter7/LConn1
